simulink model "j1tb_olctrlDemo"  (R2016b)
settings: Solver=ode5  StartTime=0.0  StopTime=inf  FixedStep=0.001  RelTol=1e-3  EnableMultiTasking=on
undefined symbols (not defined in the file): Humusoft, MF644
libraries: dcpctrl x2, sldrtlib x1, simulink x1
settings Model: SimulationMode=external  Creator=dcp  LastModifiedBy=dcp
settings OptimizationCC: LifeSpan=inf
settings DebuggingCC: SFUnexpectedBacktrackingDiag=warning  SFNoUnconditionalDefaultTransitionDiag=warning  SFExecutionAtInitializationDiag=none
settings HardwareCC: ProdBitPerLong=64  ProdHWDeviceType=Intel->x86-64 (Mac OS X)  TargetBitPerLong=64  TargetBitPerPointer=64  TargetIntDivRoundTo=Zero  TargetEndianess=LittleEndian  TargetWordSize=64  TargetHWDeviceType=Intel->x86-64
settings RTWCC: SystemTargetFile=sldrt.tlc  TemplateMakefile=sldrt.tmf  Description=Simulink Desktop Real-Time  RTWCompilerOptimization=on
settings CodeAppCC: MaxIdLength=95
settings SimulinkDesktopRealTimeCC: TargetPreCompLibLocation=/Applications/MATLAB_R2016b.app/toolbox/sldrt/lib/maci64  TargetLangStandard=C89/C90 (ANSI)  SupportVariableSizeSignals=off
settings ConfigComp: CovMetricSettings=dw  CovHtmlReporting=on  CovSaveCumulativeToWorkspaceVar=on  CovSaveSingleToWorkspaceVar=on  CovExternalEMLEnable=off

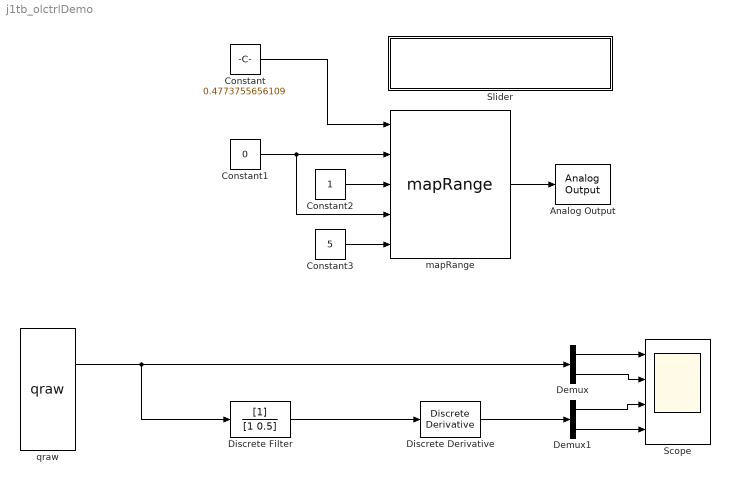
== system j1tb_olctrlDemo ==
  Analog Output : sldrtlib/Analog Output  SampleTime=0.1  MaxMissedTicks=10  ShowMissedTicks=off  YieldWhenWaiting=off  DrvName=Humusoft/MF644  DrvAddress=4294967295  DrvOptions=585  Channels=1  RangeMode=1  VoltRange=1  InitialValue=[]  FinalValue=[]
      settings: AttributesFormatString=Humusoft\nMF644 [auto]
  Constant : Constant  Value=0.4773755656109
  Constant1 : Constant  Value=0
  Constant2 : Constant
  Constant3 : Constant  Value=5
  Demux : Demux  Outputs=2
  Demux1 : Demux  Outputs=2
  Discrete Derivative : simulink/Discrete/Discrete Derivative  gainval=1.0  ICPrevScaledInput=0.0  OutMin=[]  OutMax=[]  OutDataType=fixdt(1, 16)  OutScaling=2^-10  DoSatur=off
  Discrete Filter : DiscreteFilter
  Scope : Scope  NumInputPorts=4
  Slider : Subsystem  DialogController=hmiCreateDDGDialog  IsWebBlock=on  mask(MWDashboardBlock){webBlockId=00fcefcf-6533-402e-b302-00448f9346d8, webBlockType=slider, ShowInLibBrowser=on, ShowInitialText=on, HMISrcModelName=j1testbenchctrlDemo}
      mask prompts: webBlockId "WebBlock Id"; webBlockType "WebBlock Type"; HMISrcModelName "Source Model"
      mask help: SimulinkHMI:dialogs:SliderDialogDesc
      mask Help: helpview([docroot '/mapfiles/simulink.map'], 'hmi_slider')
      mask Display:
      | if strcmp(get_param(bdroot(gcb),'BlockDiagramType'), 'library')
      |     image([(matlabroot) '/toolbox/simulink/hmi/icons/Slider.png']);
      | end
  "mapRange " : dcpctrl/mapRange 
  qraw : dcpctrl/qraw
  wires:
  "mapRange "/1 -> Analog Output/1
  Constant/1 -> "mapRange "/1
  Constant1/1 -> "mapRange "/2, "mapRange "/4
  Constant2/1 -> "mapRange "/3
  Constant3/1 -> "mapRange "/5
  qraw/2 -> Discrete Filter/1, Demux/1
  Demux/1 -> Scope/1
  Demux1/1 -> Scope/3
  Demux/2 -> Scope/2
  Demux1/2 -> Scope/4
  Discrete Filter/1 -> Discrete Derivative/1
  Discrete Derivative/1 -> Demux1/1

== system j1tb_olctrlDemo/Slider ==
